simulink model "usingSfun_speedLimiter"  (R2018b)
settings: Solver=FixedStepDiscrete  StartTime=0.0  StopTime=60  RelTol=1e-3
undefined symbols (not defined in the file): sigbuilder_block
settings Model: Creator=jlesage  LastModifiedBy=jlesage
settings SFSimCC: SimCustomHeaderCode="#include \"speedLimiter.h\""  SimUserSources=speedLimiter.c  SimAnalyzeCustomCode=on

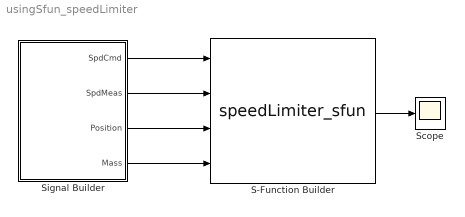
== system usingSfun_speedLimiter ==
  S-Function Builder : S-Function  InitFcn=try, set_param(gcb,'FunctionName','speedLimiter_sfun'), end  FunctionName=speedLimiter_sfun  SFunctionModules=speedLimiter_sfun_wrapper speedLimiter  SFunctionDeploymentMode=off  EnableBusSupport=off  mask(S-Function Builder){}
      mask help: Simulink:masks:SFunctionBuilder_MD
      mask init:
      | val = [[.9  0.75 0.75 1 1 .9 .9 1]',[1 1 0.75 0.75 .9 .9 1 .9]'];try , sys = get_param(gcb,'SfunBuilderFcnName');if isempty(sys), sys = get_param(gcb,'FunctionName'); end,catch, sys = get_param(gcb,'FunctionName'); end
      settings: CopyFcn=set_param(gcbh,'LinkStatus','none')  PreSaveFcn=try, set_param(gcb,'FunctionName','speedLimiter_sfun'), end  OpenFcn=sfunctionwizard(gcbh)
      mask Display: plot(val(:,1),val(:,2)),disp(sys), port_label('input',1,'spdCmd'), port_label('input',2,'spdMeas'), port_label('input',3,'x'), port_label('input',4,'m'), port_label('output',1,'spdRef')
  Scope : Scope
  Signal Builder : Subsystem  Tag=STV Subsys  LoadFcn=sigbuilder_block('load');  StartFcn=sigbuilder_block('start');  StopFcn=sigbuilder_block('stop');  ClipboardFcn=sigbuilder_block('clipboard');  mask(Sigbuilder block){tuvar=[0:10]}
      mask help: Simulink:masks:SigbuilderBlock_MD
      mask init:
      | if ~strcmp(get_param(bdroot(gcbh),'SimulationStatus'),'stopped') tuvar = sigbuilder_block('maskInit'); end
      settings: CopyFcn=sigbuilder_block('copy');  DeleteFcn=sigbuilder_block('delete');  ModelCloseFcn=sigbuilder_block('modelClose');  PreSaveFcn=sigbuilder_block('preSave');  PauseFcn=sigbuilder_block('pause');  ContinueFcn=sigbuilder_block('continue');  NameChangeFcn=sigbuilder_block('namechange');  OpenFcn=sigbuilder_block('open',[813 145.5 550.5 399.75 ]);  CloseFcn=sigbuilder_block('close');
      mask Display: plot(0, 0, 100, 100,[2, 2, 32, 32, 2], [68, 8, 8, 68, 68],[32, 2], [38, 38], [32, 19, 2],[53, 60, 44], [32, 17, 17, 2],[16, 16, 31, 31]);txt = getActiveGroup(gcbh);text(2, 100, txt,'verticalAlignment', 'top');
  wires:
  S-Function Builder/1 -> Scope/1
  Signal Builder/1(SpdCmd) -> S-Function Builder/1
  Signal Builder/2(SpdMeas) -> S-Function Builder/2
  Signal Builder/3(Position) -> S-Function Builder/3
  Signal Builder/4(Mass) -> S-Function Builder/4

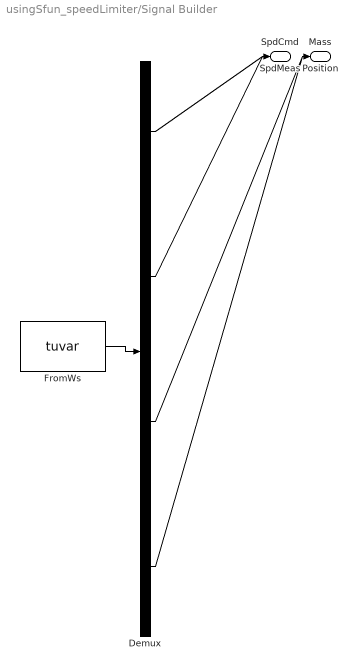
== system usingSfun_speedLimiter/Signal Builder ==
  Demux : Demux  Tag=STV Demux
  FromWs : FromWorkspace  Tag=STV FromWs  VariableName=tuvar  SampleTime=0.1
      SigBuilderData=|
      | common.afterFinalStr = 'Extrapolate'
      | common.sampleTime = '0.1'
      | dataSet(1).timeRange = [0 60]
      | dataSet(1).name = 'RaiseBlock'
      | dataSet(2).timeRange = [0 60]
      | dataSet(2).name = 'LowerBlock'
      | dataSet(3).timeRange = [0 60]
      | dataSet(3).name = 'RaiseLower'
      | sbobj.Groups(1).Name = 'RaiseBlock'
      | sbobj.Groups(1).Signals(1).Name = 'SpdCmd'
      | sbobj.Groups(1).Signals(1).XData = [0 60]
      | sbobj.Groups(1).Signals(1).YData = [1500 1500]
      | sbobj.Groups(1).Signals(2).Name = 'SpdMeas'
      | sbobj.Groups(1).Signals(2).XData = [0 60]
      | sbobj.Groups(1).Signals(2).YData = [750 750]
      | sbobj.Groups(1).Signals(3).Name = 'Position'
      | sbobj.Groups(1).Signals(3).XData = [0 1 50 60]
      | sbobj.Groups(1).Signals(3).YData = [0 0 50 50]
      | sbobj.Groups(1).Signals(4).Name = 'Mass'
      | sbobj.Groups(1).Signals(4).XData = [0 60]
      | sbobj.Groups(1).Signals(4).YData = [112500 112500]
      | sbobj.Groups(1).TimeRange = [0 60]
      | sbobj.Groups(2).Name = 'LowerBlock'
      | sbobj.Groups(2).Signals(1).Name = 'SpdCmd'
      | sbobj.Groups(2).Signals(1).XData = [0 60]
      | sbobj.Groups(2).Signals(1).YData = [-1500 -1500]
      | sbobj.Groups(2).Signals(2).Name = 'SpdMeas'
      | sbobj.Groups(2).Signals(2).XData = [0 60]
      | sbobj.Groups(2).Signals(2).YData = [-750 -750]
      | sbobj.Groups(2).Signals(3).Name = 'Position'
      | sbobj.Groups(2).Signals(3).XData = [0 1 50 60]
      | sbobj.Groups(2).Signals(3).YData = [48 48 0 0]
      | sbobj.Groups(2).Signals(4).Name = 'Mass'
      | sbobj.Groups(2).Signals(4).XData = [0 60]
      | sbobj.Groups(2).Signals(4).YData = [112500 112500]
      | sbobj.Groups(2).TimeRange = [0 60]
      | sbobj.Groups(3).Name = 'RaiseLower'
      | sbobj.Groups(3).Signals(1).Name = 'SpdCmd'
      | sbobj.Groups(3).Signals(1).XData = [0 25 25.1 30 30.1 55 55.1 60]
      | sbobj.Groups(3).Signals(1).YData = [1500 1500 0 0 -1500 -1500 0 0]
      | sbobj.Groups(3).Signals(2).Name = 'SpdMeas'
      | sbobj.Groups(3).Signals(2).XData = [0 25.1 25.1 30 30.01 60]
      | sbobj.Groups(3).Signals(2).YData = [750 750 0 0 -750 -750]
      | sbobj.Groups(3).Signals(3).Name = 'Position'
      | sbobj.Groups(3).Signals(3).XData = [0 1 25 30 55 60]
      | sbobj.Groups(3).Signals(3).YData = [0 0 50 50 0 0]
      | sbobj.Groups(3).Signals(4).Name = 'Mass'
      | sbobj.Groups(3).Signals(4).XData = [0 60]
      | sbobj.Groups(3).Signals(4).YData = [112500 112500]
      | sbobj.Groups(3).TimeRange = [0 60]
  SpdCmd : Outport  Tag=STV Outport
  SpdMeas : Outport  Tag=STV Outport  Port=2
  Position : Outport  Tag=STV Outport  Port=3
  Mass : Outport  Tag=STV Outport  Port=4
  wires:
  FromWs/1 -> Demux/1
  Demux/1 -> SpdCmd/1
  Demux/2 -> SpdMeas/1
  Demux/3 -> Position/1
  Demux/4 -> Mass/1
